simulink model "rrc_v_rect_bw"  (R2013a)
settings: Solver=ode45  StartTime=0.0  StopTime=0.5  RelTol=1e-3
libraries: dsparch4 x2, dspsigops x1
settings Model: Creator=hebin  LastModifiedBy=hebin

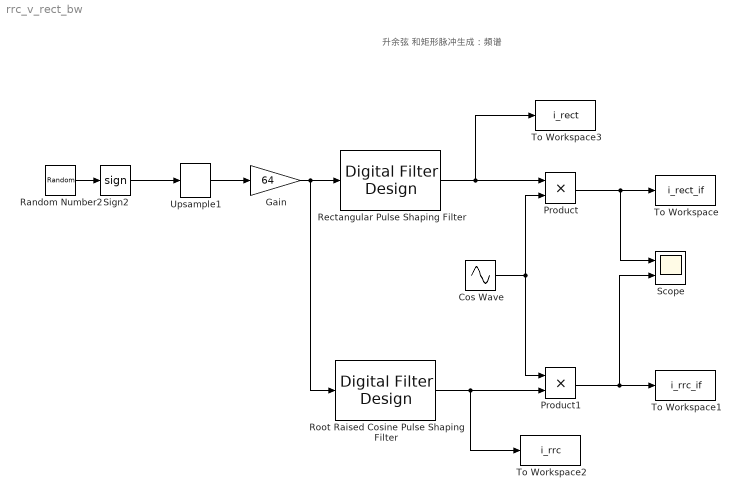
== system rrc_v_rect_bw ==
  note: 升余弦 和矩形脉冲生成：频谱
  Cos Wave : Sin  Frequency=(38.4e+3)*2*pi  Phase=pi/2  SampleTime=1/153.6e+3
  Gain : Gain  Gain=64
  Product : Product  RndMeth=Zero
  Product1 : Product  RndMeth=Zero
  Random Number2 : RandomNumber  Seed=777  SampleTime=1/2400
  Rectangular Pulse Shaping Filter : dsparch4/Digital Filter Design  mwdsp_browser_bugfix_var=off
  Root Raised Cosine Pulse Shaping Filter : dsparch4/Digital Filter Design  mwdsp_browser_bugfix_var=off
  Scope : Scope  NumInputPorts=2
      settings: YMin=-5~-5  YMax=5~5
  Sign2 : Signum
  To Workspace : ToWorkspace  VariableName=i_rect_if  SampleTime=-1
  To Workspace1 : ToWorkspace  VariableName=i_rrc_if  SampleTime=-1
  To Workspace2 : ToWorkspace  VariableName=i_rrc  SampleTime=-1
  To Workspace3 : ToWorkspace  VariableName=i_rect  SampleTime=-1
  Upsample1 : dspsigops/Upsample  N=64  phase=0  InputProcessing=Inherited (this choice will be removed - see release notes)  RateOptions=Allow multirate processing  ic=0  mode=Unused parameter value
  wires:
  Rectangular Pulse Shaping Filter/1 -> Product/1, To Workspace3/1
  Product/1 -> Scope/1, To Workspace/1
  Upsample1/1 -> Gain/1
  Cos Wave/1 -> Product/2, Product1/1
  Gain/1 -> Root Raised Cosine Pulse Shaping Filter/1, Rectangular Pulse Shaping Filter/1
  Root Raised Cosine Pulse Shaping Filter/1 -> To Workspace2/1, Product1/2
  Product1/1 -> To Workspace1/1, Scope/2
  Random Number2/1 -> Sign2/1
  Sign2/1 -> Upsample1/1
